simulink model "train_model_nika"  (R2021b)
settings: Solver=ode4  StartTime=0.0  StopTime=10  FixedStep=0.01  RelTol=1e-3
undefined symbols (not defined in the file): g, l
libraries: simulink_extras x1
settings Model: Creator=mlx-0  LastModifiedBy=Acer

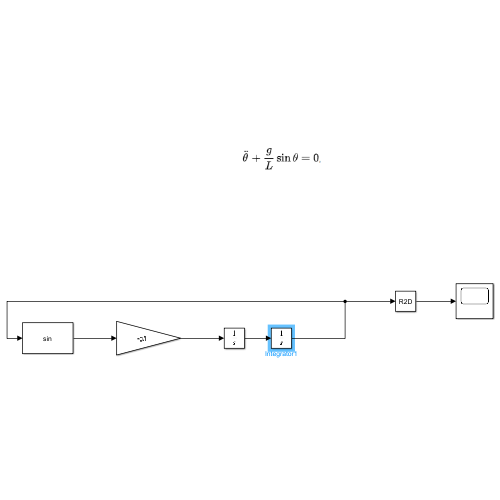
[thumbnail: Simulink's stored preview of the top-level diagram]
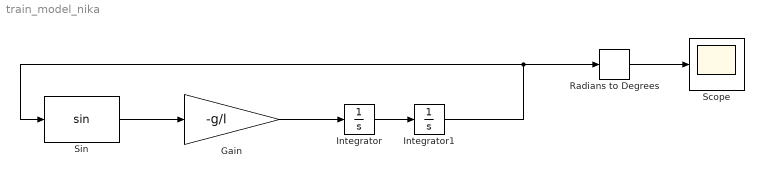
== system train_model_nika ==
  Gain : Gain  Gain=-g/l
  Integrator : Integrator
  Integrator1 : Integrator
  Radians to Degrees : simulink_extras/Transformations/Radians to Degrees
  Scope : Scope
  Sin : Trigonometry
  wires:
  Sin/1 -> Gain/1
  Gain/1 -> Integrator/1
  Integrator1/1 -> Radians to Degrees/1, Sin/1
  Radians to Degrees/1 -> Scope/1
  Integrator/1 -> Integrator1/1
